simulink model "Nadir_Pointing"  (R2023b)
settings: Solver=VariableStepAuto  StartTime=0.0  StopTime=10.0  RelTol=1e-3
values from neighbouring files (symbols this model uses):
  a = 7259    [Group_51.m]
  a_sun = 149.60e6    (= 149600000)    [Group_51.m]
  ARW = (((arw*pi/180)/(sqrt(n_t)))^2)*n_t    [Group_51.m]
  Beta_CMG = acos(dot([1;0;0],uv_pyr))    [Group_51.m]
  delta_0_P = SM.delta_g_SM(end,:)    [Group_51.m]
  e = 0.001    [Group_51.m]
  e_sun = 0.0167086    [Group_51.m]
  eps_b = 11.5*pi/180    (= 0.200712863979)    [Group_51.m]
  eps_sun = deg2rad(23.45)    [Group_51.m]
  f0_P = SM.Theta_SM(end,1)    [Group_51.m]
  g_1_0 = -29404.8    [Group_51.m]
  g_1_1 = -1450.9    [Group_51.m]
  Gain_G = eye(3,3)    [Group_51.m]
  h_1_1 = 4653.5    [Group_51.m]
  h_r = [0.5;0.5;0.5;0.5]    [Group_51.m]
  halfrange = pi/40    (= 0.0785398163397)    [Group_51.m]
  i = deg2rad(97.27276)    [Group_51.m]
  I_tot = I+Ip_1_transp+Ip_2_transp    [Group_51.m]
  I_tot_inv = I_tot\eye(3,3)    [Group_51.m]
  IC312_P = [phi312_P;theta312_P;psi312_P]    [Group_51.m]
  jb = [0.1; 0.1;0.1]    [Group_51.m]
  k_cmg = -1    [Group_51.m]
  kdx_P = 2    [Group_51.m]
  kdy_P = 2.365    [Group_51.m]
  kdz_P = 2.1    [Group_51.m]
  kpx_SM = 0.129*0.5    (= 0.0645)    [Group_51.m]
  kpy_P = 1.4*0.5    (= 0.7)    [Group_51.m]
  kpz_P = 1*0.5    (= 0.5)    [Group_51.m]
  Miss_G = [teta_g_x;teta_g_y;teta_g_z]    [Group_51.m]
  n = sqrt(mu/ a^3)    [Group_51.m]
  n_sun = 2*pi/(365.26*24*3600)    (= 1.99096676796e-07)    [Group_51.m]
  n_t = samp_t    (= 1)    [Group_51.m]
  OM = deg2rad(90)    [Group_51.m]
  Re = astroConstants(23)    [Group_51.m]
  RRW = (((rrw*pi/180)/(sqrt(n_t)))^2)*n_t    [Group_51.m]
  samp_t = 1/samp_freq    (= 1)    [Group_51.m]
  t_sun_P = tf_D+tf_SM    (= 550)    [Group_51.m]
  w = deg2rad(0)    [Group_51.m]
  w0_P = [wx_P;wy_P;wz_P]    [Group_51.m]
  we = we/3600    (= 7.29159776389e-06)    [Group_51.m]
undefined symbols (not defined in the file or in its folder): DiscIntNeverNeededParam
libraries: matrix_library x15, vrlib x11, simulink x6, hdlsllib x2, dspswit3 x1
(part 1 of 2)
settings Model: Creator=leo-deo  LastModifiedBy=leo-deo

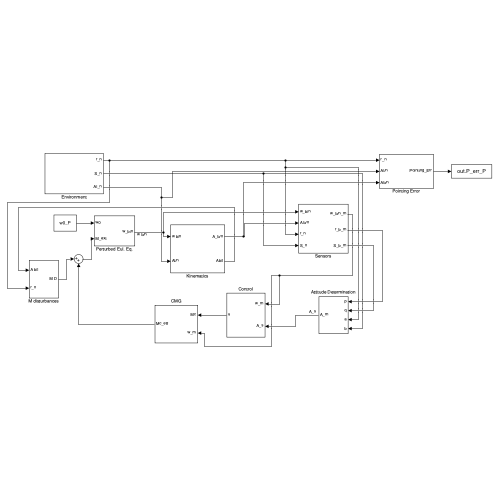
[thumbnail: Simulink's stored preview of the top-level diagram]
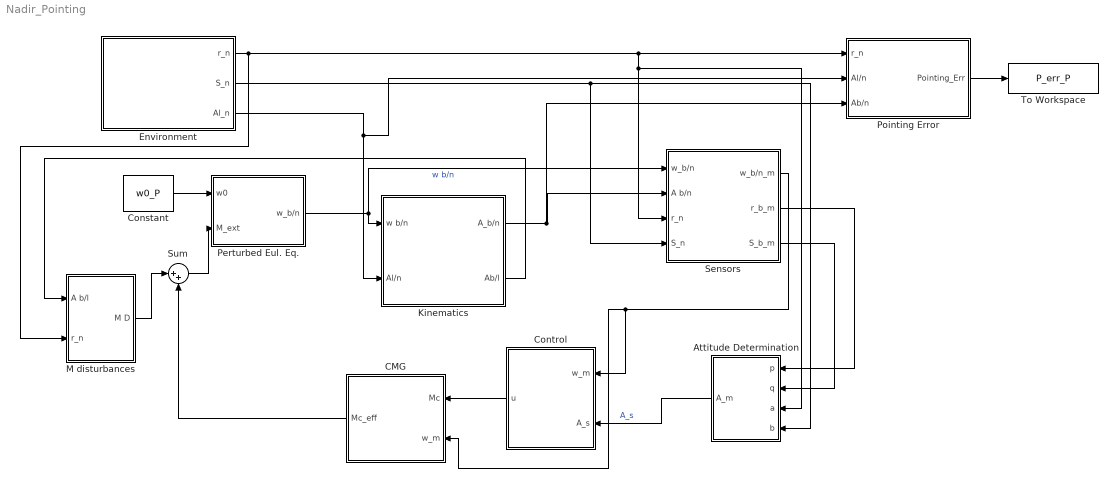
== system Nadir_Pointing ==
  Attitude Determination : Subsystem
  CMG : Subsystem
  Constant : Constant  Value=w0_P
  Control : Subsystem
  Environment : Subsystem
  Kinematics : Subsystem
  M disturbances : Subsystem
  Perturbed Eul. Eq. : Subsystem
  Pointing Error : Subsystem
  Sensors : Subsystem
  Sum : Sum  Inputs=|++
  To Workspace : ToWorkspace  VariableName=P_err_P  SampleTime=-1
  wires:
  M disturbances/1(M D) -> Sum/1
  Sensors/3(S_b_m) -> Attitude Determination/2(q)
  Kinematics/2(Ab/l) -> M disturbances/1(A b/l)
  Environment/2(S_n) -> Attitude Determination/4(b), Sensors/4(S_n)
  Sensors/1(w_b/n_m) -> Control/1(w_m), CMG/2(w_m)
  Kinematics/1(A_b/n) -> Pointing Error/3(Ab/n), Sensors/2(A b/n)
  Perturbed Eul. Eq./1(w_b/n) -> Sensors/1(w_b/n), Kinematics/1(w b/n)  "w b/n"
  Environment/3(Al_n) -> Pointing Error/2(Al/n), Kinematics/2(Al/n)
  Sum/1 -> Perturbed Eul. Eq./2(M_ext)
  Sensors/2(r_b_m) -> Attitude Determination/1(p)
  Constant/1 -> Perturbed Eul. Eq./1(w0)
  CMG/1(Mc_eff) -> Sum/2
  Control/1(u) -> CMG/1(Mc)
  Environment/1(r_n) -> M disturbances/2(r_n), Pointing Error/1(r_n), Attitude Determination/3(a), Sensors/3(r_n)
  Attitude Determination/1(A_m) -> Control/2(A_s)  "A_s"
  Pointing Error/1(Pointing_Err) -> To Workspace/1

== system Nadir_Pointing/Attitude Determination ==
  p : Inport
  q : Inport  Port=2
  a : Inport  Port=3
  b : Inport  Port=4
  Cross Product{,1..3} (4 alike) : matrix_library/Cross Product
  Matrix Concatenate : Concatenate  NumInputs=3  Mode=Multidimensional array  ConcatenateDimension=2
  Matrix Concatenate1 : Concatenate  NumInputs=3  Mode=Multidimensional array  ConcatenateDimension=2
  Normalize Vector{,1..5} (6 alike) : vrlib/Utilities/Normalize Vector  maxzero=0
  Product : Product  Multiplication=Matrix(*)
  Transpose : Math  Operator=transpose
  Zero-Order Hold : ZeroOrderHold  SampleTime=samp_t
  Zero-Order Hold1 : ZeroOrderHold  SampleTime=samp_t
  A_m : Outport
  wires:
  Matrix Concatenate1/1 -> Transpose/1
  Cross Product/1 -> Normalize Vector4/1
  Normalize Vector3/1 -> Matrix Concatenate1/3  "v3"
  Cross Product3/1 -> Normalize Vector3/1
  Product/1 -> A_m/1
  Cross Product1/1 -> Normalize Vector5/1
  Transpose/1 -> Product/2
  Matrix Concatenate/1 -> Product/1
  Normalize Vector2/1 -> Matrix Concatenate1/2, Cross Product3/2  "v2"
  Normalize Vector4/1 -> Matrix Concatenate/2, Cross Product1/2  "s2"
  q/1 -> Cross Product/2
  Cross Product2/1 -> Normalize Vector2/1
  p/1 -> Cross Product/1, Matrix Concatenate/1, Cross Product1/1  "s1"
  a/1 -> Zero-Order Hold/1
  Normalize Vector/1 -> Matrix Concatenate1/1, Cross Product3/1, Cross Product2/1  "v1"
  b/1 -> Zero-Order Hold1/1
  Normalize Vector1/1 -> Cross Product2/2
  Zero-Order Hold/1 -> Normalize Vector/1
  Zero-Order Hold1/1 -> Normalize Vector1/1
  Normalize Vector5/1 -> Matrix Concatenate/3

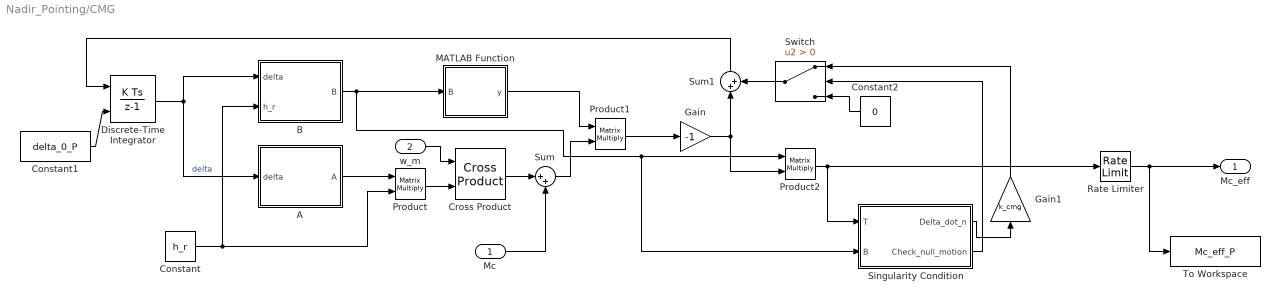
== system Nadir_Pointing/CMG ==
  Mc : Inport
  w_m : Inport  Port=2
  A : Subsystem
  B : Subsystem
  Constant : Constant  Value=h_r
  Constant1 : Constant  Value=delta_0_P
  Constant2 : Constant  Value=0
  Cross Product : matrix_library/Cross Product
  Discrete-Time Integrator : DiscreteIntegrator  InitialConditionSource=external  SampleTime=-1  ICPrevOutput=DiscIntNeverNeededParam  ICPrevScaledInput=DiscIntNeverNeededParam
  Gain : Gain  Gain=-1
  Gain1 : Gain  Gain=k_cmg
  MATLAB Function : MATLAB Function  TreatAsAtomicUnit=on
  Product : Product  Multiplication=Matrix(*)
  Product1 : Product  Multiplication=Matrix(*)
  Product2 : Product  Multiplication=Matrix(*)
  Rate Limiter : RateLimiter  RisingSlewLimit=samp_t  FallingSlewLimit=-samp_t
  Singularity Condition : Subsystem
  Sum : Sum  Inputs=|++
  Sum1 : Sum  Inputs=|++
  Switch : Switch  Criteria=u2 > Threshold  SaturateOnIntegerOverflow=off  InputSameDT=off
  To Workspace : ToWorkspace  VariableName=Mc_eff_P  SampleTime=-1
  Mc_eff : Outport
  wires:
  Rate Limiter/1 -> To Workspace/1, Mc_eff/1
  MATLAB Function/1(y) -> Product1/1
  Discrete-Time Integrator/1 -> B/1(delta), A/1(delta)  "delta"
  w_m/1 -> Cross Product/1
  Cross Product/1 -> Sum/1
  Sum/1 -> Product1/2
  Product1/1 -> Gain/1
  Constant/1 -> B/2(h_r), Product/2
  B/1(B) -> MATLAB Function/1(B), Singularity Condition/2(B), Product2/1
  Product/1 -> Cross Product/2
  A/1(A) -> Product/1
  Gain/1 -> Sum1/1, Product2/2
  Constant1/1 -> Discrete-Time Integrator/2
  Product2/1 -> Rate Limiter/1, Singularity Condition/1(T)
  Sum1/1 -> Discrete-Time Integrator/1
  Switch/1 -> Sum1/2
  Constant2/1 -> Switch/3
  Singularity Condition/2(Check_null_motion) -> Switch/2
  Mc/1 -> Sum/2
  Singularity Condition/1(Delta_dot_n) -> Gain1/1
  Gain1/1 -> Switch/1

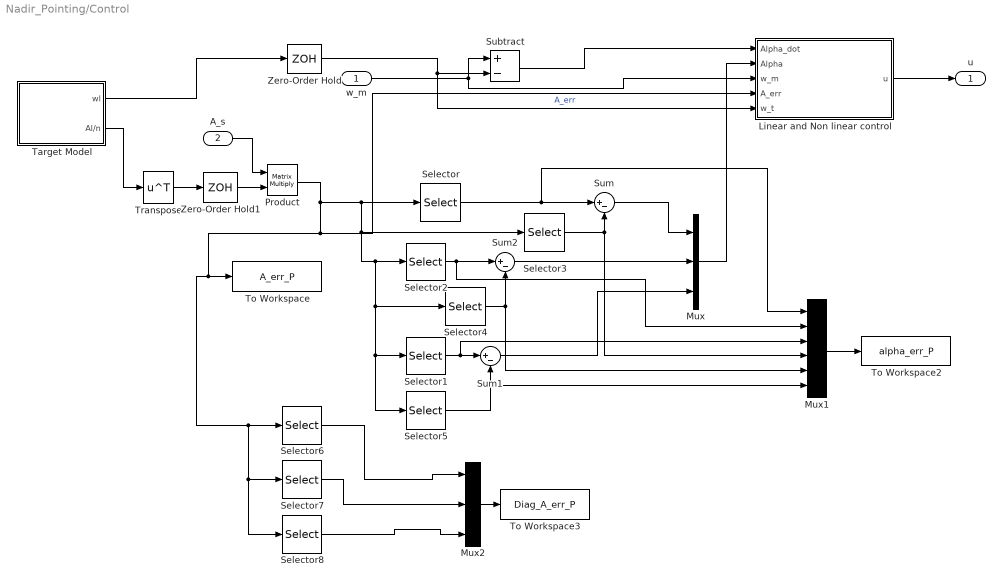
== system Nadir_Pointing/Control ==
  w_m : Inport
  A_s : Inport  Port=2
  Linear and Non linear control : Subsystem
  Mux : Mux  Inputs=3
  Mux1 : Mux  Inputs=6
  Mux2 : Mux  Inputs=3
  Product : Product  Multiplication=Matrix(*)
  Selector : Selector  NumberOfDimensions=2  InputPortWidth=3  IndexOptions=Index vector (dialog),Index vector (dialog)  Indices=2,3  OutputSizes=1,1
  Selector1 : Selector  NumberOfDimensions=2  InputPortWidth=3  IndexOptions=Index vector (dialog),Index vector (dialog)  Indices=1,2  OutputSizes=1,1
  Selector2 : Selector  NumberOfDimensions=2  InputPortWidth=3  IndexOptions=Index vector (dialog),Index vector (dialog)  Indices=3,1  OutputSizes=1,1
  Selector3 : Selector  NumberOfDimensions=2  InputPortWidth=3  IndexOptions=Index vector (dialog),Index vector (dialog)  Indices=3,2  OutputSizes=1,1
  Selector4 : Selector  NumberOfDimensions=2  InputPortWidth=3  IndexOptions=Index vector (dialog),Index vector (dialog)  Indices=1,3  OutputSizes=1,1
  Selector5 : Selector  NumberOfDimensions=2  InputPortWidth=3  IndexOptions=Index vector (dialog),Index vector (dialog)  Indices=2,1  OutputSizes=1,1
  Selector6 : Selector  NumberOfDimensions=2  InputPortWidth=3  IndexOptions=Index vector (dialog),Index vector (dialog)  Indices=1,1  OutputSizes=1,1
  Selector7 : Selector  NumberOfDimensions=2  InputPortWidth=3  IndexOptions=Index vector (dialog),Index vector (dialog)  Indices=2,2  OutputSizes=1,1
  Selector8 : Selector  NumberOfDimensions=2  InputPortWidth=3  IndexOptions=Index vector (dialog),Index vector (dialog)  Indices=3,3  OutputSizes=1,1
  Subtract : Sum  Inputs=+-
  Sum : Sum  Inputs=|+-
  Sum1 : Sum  Inputs=|+-
  Sum2 : Sum  Inputs=|+-
  Target Model : Subsystem
  To Workspace : ToWorkspace  VariableName=A_err_P  SampleTime=-1
  To Workspace2 : ToWorkspace  VariableName=alpha_err_P  SampleTime=-1
  To Workspace3 : ToWorkspace  VariableName=Diag_A_err_P  SampleTime=-1
  Transpose : Math  Operator=transpose
  Zero-Order Hold : ZeroOrderHold  SampleTime=samp_t
  Zero-Order Hold1 : ZeroOrderHold  SampleTime=samp_t
  u : Outport
  wires:
  A_s/1 -> Product/1
  Target Model/2(Al/n) -> Transpose/1
  Subtract/1 -> Linear and Non linear control/1(Alpha_dot)
  w_m/1 -> Linear and Non linear control/3(w_m), Subtract/1
  Product/1 -> Selector3/1, Selector4/1, Selector5/1, Selector1/1, Selector2/1, Selector/1, To Workspace/1, Selector8/1, Selector7/1, Selector6/1, Linear and Non linear control/4(A_err)  "A_err"
  Linear and Non linear control/1(u) -> u/1
  Selector/1 -> Mux1/1, Sum/1
  Selector2/1 -> Mux1/2, Sum2/1
  Selector1/1 -> Mux1/3, Sum1/1
  Selector3/1 -> Mux1/4, Sum/2
  Sum/1 -> Mux/1
  Mux/1 -> Linear and Non linear control/2(Alpha)
  Selector4/1 -> Sum2/2, Mux1/5
  Sum2/1 -> Mux/2
  Selector5/1 -> Mux1/6, Sum1/2
  Sum1/1 -> Mux/3
  Mux1/1 -> To Workspace2/1
  Transpose/1 -> Zero-Order Hold1/1
  Selector7/1 -> Mux2/2
  Selector8/1 -> Mux2/3
  Mux2/1 -> To Workspace3/1
  Selector6/1 -> Mux2/1
  Target Model/1(wl) -> Zero-Order Hold/1
  Zero-Order Hold/1 -> Linear and Non linear control/5(w_t), Subtract/2
  Zero-Order Hold1/1 -> Product/2

== system Nadir_Pointing/Environment ==
  A l/n for elliptical orbit : Subsystem
  Clock : Clock
  Kep 2bp : Subsystem
  "Sn " : Subsystem
  To Workspace : ToWorkspace  VariableName=t_P  SampleTime=-1
  r_n : Outport
  S_n : Outport  Port=2
  Al_n : Outport  Port=3
  wires:
  Kep 2bp/1(r_n) -> r_n/1
  "Sn "/1(Sn) -> S_n/1
  A l/n for elliptical orbit/1(Al/n) -> Al_n/1
  Clock/1 -> To Workspace/1
  A l/n for elliptical orbit/2(Theta) -> Kep 2bp/1(Theta)

== system Nadir_Pointing/Kinematics ==
  w b/n : Inport
  Al/n : Inport  Port=2
  Euler Angles : Subsystem
  Product2 : Product  Multiplication=Matrix(*)
  Subsystem : Subsystem
  To Workspace : ToWorkspace  VariableName=A_bn_P  SampleTime=-1
  Transpose1 : Math  Operator=transpose
  A_b/n : Outport
  Ab/l : Outport  Port=2
  wires:
  w b/n/1 -> Euler Angles/1(w_b)
  Al/n/1 -> Transpose1/1
  Transpose1/1 -> Product2/2
  Product2/1 -> Ab/l/1  "Ab/l"
  Euler Angles/1(A_b/n) -> Product2/1, To Workspace/1, A_b/n/1
  Euler Angles/2(Ang_312) -> Subsystem/1(Ang_312)
  Euler Angles/3(Ang_313) -> Subsystem/2(Ang_313)
  Euler Angles/4(T-F) -> Subsystem/3(T-F)

== system Nadir_Pointing/M disturbances ==
  A b/l : Inport
  r_n : Inport  Port=2
  M of B : Subsystem
  M of G G : Subsystem
  Sum : Sum  Inputs=||+||+||
  M D : Outport
  wires:
  Sum/1 -> M D/1
  A b/l/1 -> M of B/1(A b/n), M of G G/1(Ab/l)
  M of G G/1(M_G_G) -> Sum/2
  M of B/1(M B) -> Sum/1
  r_n/1 -> M of B/2(r_n)

== system Nadir_Pointing/Perturbed Eul. Eq. ==
  w0 : Inport
  M_ext : Inport  Port=2
  Constant2 : Constant  Value=I_tot
  Constant3 : Constant  Value=I_tot_inv
  Cross Product : matrix_library/Cross Product
  Integrator1 : Integrator  InitialConditionSource=external  AbsoluteTolerance=1e-10
  Product : Product  Multiplication=Matrix(*)
  Product1 : Product  Multiplication=Matrix(*)
  Product2 : Product  Multiplication=Matrix(*)
  Sum : Sum  Inputs=|-+
  To Workspace : ToWorkspace  VariableName=w_b_P  SampleTime=-1
  w_b/n : Outport
  wires:
  Constant2/1 -> Product/1
  Product/1 -> Cross Product/2
  Product2/1 -> Sum/2
  Sum/1 -> Integrator1/1
  Constant3/1 -> Product2/1, Product1/1
  Cross Product/1 -> Product1/2
  Integrator1/1 -> Cross Product/1, Product/2, To Workspace/1, w_b/n/1
  Product1/1 -> Sum/1
  w0/1 -> Integrator1/2
  M_ext/1 -> Product2/2

== system Nadir_Pointing/Pointing Error ==
  r_n : Inport
  Al/n : Inport  Port=2
  Ab/n : Inport  Port=3
  Acos : Trigonometry  Operator=acos
  Dot Product : DotProduct  OutDataTypeStr=Inherit: Inherit via internal rule
  Normalize Vector : vrlib/Utilities/Normalize Vector  maxzero=0
  Normalize Vector1 : vrlib/Utilities/Normalize Vector  maxzero=0
  Product : Product  Multiplication=Matrix(*)
  Product1 : Product  Multiplication=Matrix(*)
  Scope : Scope
  Pointing_Err : Outport
  wires:
  Ab/n/1 -> Product1/1
  Al/n/1 -> Product/1
  Normalize Vector/1 -> Dot Product/2
  Product1/1 -> Normalize Vector/1
  Dot Product/1 -> Acos/1
  r_n/1 -> Product/2, Product1/2
  Normalize Vector1/1 -> Dot Product/1
  Product/1 -> Normalize Vector1/1
  Acos/1 -> Scope/1, Pointing_Err/1

== system Nadir_Pointing/Sensors ==
  w_b/n : Inport
  A b/n : Inport  Port=2
  r_n : Inport  Port=3
  S_n : Inport  Port=4
  Clock : Clock
  Gyroscopic Sensor : Subsystem
  Horizon Sensor1 : Subsystem
  Normalize Vector : vrlib/Utilities/Normalize Vector  maxzero=0
  Normalize Vector1 : vrlib/Utilities/Normalize Vector  maxzero=0
  Product : Product  Multiplication=Matrix(*)
  Product1 : Product  Multiplication=Matrix(*)
  Sun Sensor1 : Subsystem
  To Workspace : ToWorkspace  VariableName=t_s_P  SampleTime=-1
  Zero-Order Hold : ZeroOrderHold  SampleTime=samp_t
  w_b/n_m : Outport
  r_b_m : Outport  Port=2
  S_b_m : Outport  Port=3
  wires:
  S_n/1 -> Product1/2
  Product/1 -> Normalize Vector/1
  A b/n/1 -> Product/1, Product1/1
  r_n/1 -> Product/2
  w_b/n/1 -> Gyroscopic Sensor/1(w_b/n)
  Sun Sensor1/1(S_b_m) -> S_b_m/1  "s3"
  Normalize Vector1/1 -> Sun Sensor1/1(S_b)  "s3"
  Product1/1 -> Normalize Vector1/1
  Gyroscopic Sensor/1(w_b/n_m) -> w_b/n_m/1
  Normalize Vector/1 -> Horizon Sensor1/1(r_b)  "s3"
  Horizon Sensor1/1(r_b_m) -> r_b_m/1  "s3"
  Clock/1 -> Zero-Order Hold/1
  Zero-Order Hold/1 -> To Workspace/1

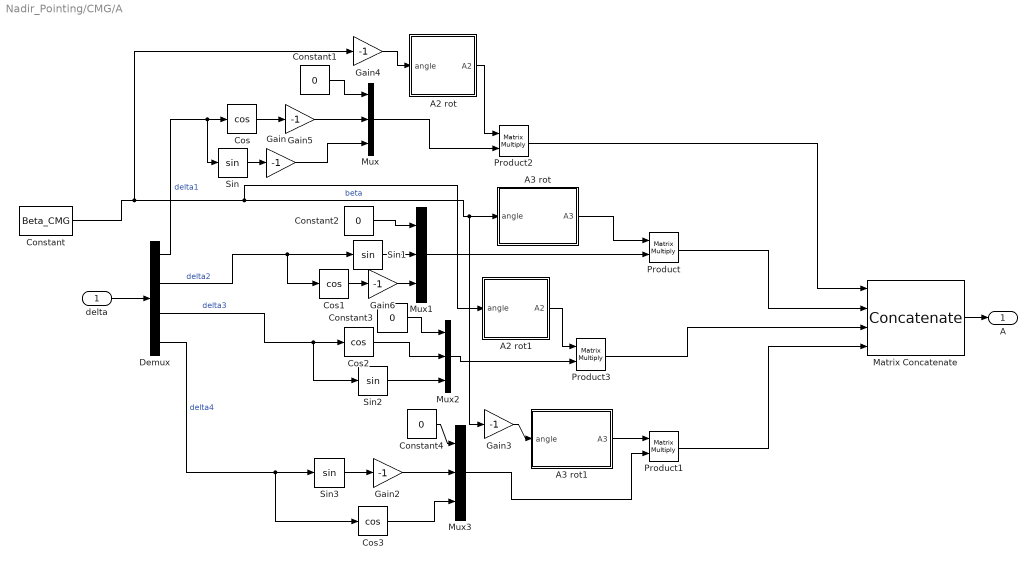
== system Nadir_Pointing/CMG/A ==
  delta : Inport
  A2 rot : Subsystem
  A2 rot1 : Subsystem
  A3 rot : Subsystem
  A3 rot1 : Subsystem
  Constant : Constant  Value=Beta_CMG
  Constant{1..4} (4 alike) : Constant  Value=0
  Cos{,1..3} (4 alike) : Trigonometry  Operator=cos
  Demux : Demux
  Gain{,2..6} (6 alike) : Gain  Gain=-1
  Matrix Concatenate : Concatenate  NumInputs=4  Mode=Multidimensional array  ConcatenateDimension=2
  Mux{,1..3} (4 alike) : Mux  Inputs=3
  Product{,1..3} (4 alike) : Product  Multiplication=Matrix(*)
  Sin{,1..3} (4 alike) : Trigonometry
  A : Outport
  wires:
  Constant4/1 -> Mux3/1
  Constant2/1 -> Mux1/1
  Sin3/1 -> Gain2/1
  Sin/1 -> Gain/1
  delta/1 -> Demux/1
  Demux/1 -> Sin/1, Cos/1  "delta1"
  Gain/1 -> Mux/3
  Constant1/1 -> Mux/1
  Constant3/1 -> Mux2/1
  Sin1/1 -> Mux1/2
  Demux/2 -> Cos1/1, Sin1/1  "delta2"
  Cos3/1 -> Mux3/3
  Gain2/1 -> Mux3/2
  Demux/4 -> Cos3/1, Sin3/1  "delta4"
  Mux1/1 -> Product/2
  Constant/1 -> Gain4/1, A2 rot1/1(angle), Gain3/1, A3 rot/1(angle)  "beta"
  A3 rot/1(A3) -> Product/1
  Product/1 -> Matrix Concatenate/2
  Gain3/1 -> A3 rot1/1(angle)
  A3 rot1/1(A3) -> Product1/1
  Mux3/1 -> Product1/2
  Product1/1 -> Matrix Concatenate/4
  A2 rot/1(A2) -> Product2/1
  Mux/1 -> Product2/2
  Gain4/1 -> A2 rot/1(angle)
  Product2/1 -> Matrix Concatenate/1
  Mux2/1 -> Product3/2
  Product3/1 -> Matrix Concatenate/3
  A2 rot1/1(A2) -> Product3/1
  Matrix Concatenate/1 -> A/1
  Gain5/1 -> Mux/2
  Cos/1 -> Gain5/1
  Gain6/1 -> Mux1/3
  Cos1/1 -> Gain6/1
  Sin2/1 -> Mux2/3
  Cos2/1 -> Mux2/2
  Demux/3 -> Sin2/1, Cos2/1  "delta3"

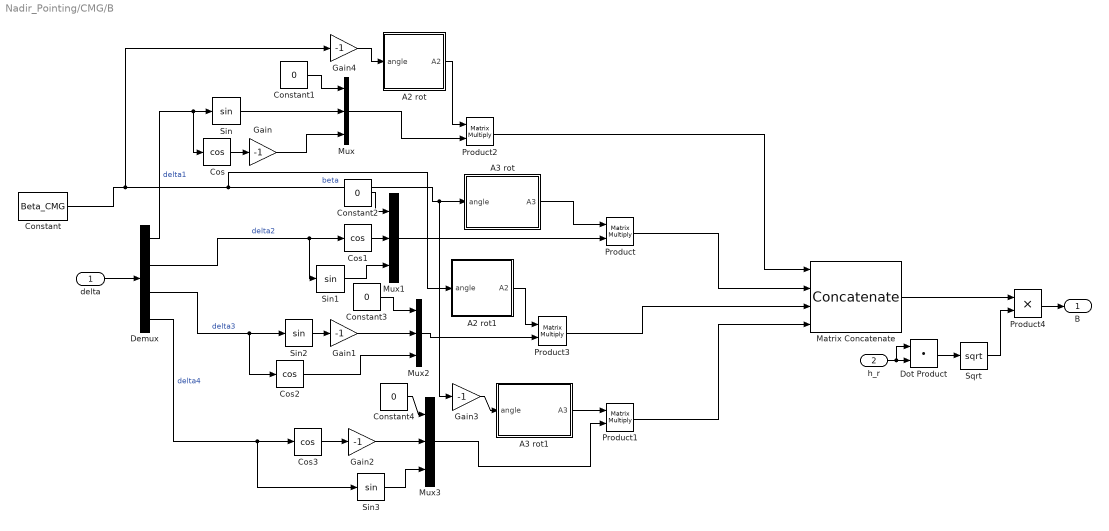
== system Nadir_Pointing/CMG/B ==
  delta : Inport
  h_r : Inport  Port=2
  A2 rot : Subsystem
  A2 rot1 : Subsystem
  A3 rot : Subsystem
  A3 rot1 : Subsystem
  Constant : Constant  Value=Beta_CMG
  Constant{1..4} (4 alike) : Constant  Value=0
  Cos{,1..3} (4 alike) : Trigonometry  Operator=cos
  Demux : Demux
  Dot Product : DotProduct  OutDataTypeStr=Inherit: Inherit via internal rule
  Gain{,1..4} (5 alike) : Gain  Gain=-1
  Matrix Concatenate : Concatenate  NumInputs=4  Mode=Multidimensional array  ConcatenateDimension=2
  Mux{,1..3} (4 alike) : Mux  Inputs=3
  Product{,1..3} (4 alike) : Product  Multiplication=Matrix(*)
  Product4 : Product
  Sin{,1..3} (4 alike) : Trigonometry
  Sqrt : Sqrt
  B : Outport
  wires:
  Constant4/1 -> Mux3/1
  Sin1/1 -> Mux1/3
  Constant2/1 -> Mux1/1
  Cos3/1 -> Gain2/1
  Cos/1 -> Gain/1
  delta/1 -> Demux/1
  Demux/1 -> Cos/1, Sin/1  "delta1"
  Gain/1 -> Mux/3
  Gain1/1 -> Mux2/2
  Constant1/1 -> Mux/1
  Constant3/1 -> Mux2/1
  Cos1/1 -> Mux1/2
  Demux/2 -> Cos1/1, Sin1/1  "delta2"
  Sin3/1 -> Mux3/3
  Cos2/1 -> Mux2/3
  Gain2/1 -> Mux3/2
  Sin/1 -> Mux/2
  Demux/4 -> Sin3/1, Cos3/1  "delta4"
  Sin2/1 -> Gain1/1
  Demux/3 -> Cos2/1, Sin2/1  "delta3"
  Mux1/1 -> Product/2
  Constant/1 -> Gain4/1, A2 rot1/1(angle), Gain3/1, A3 rot/1(angle)  "beta"
  A3 rot/1(A3) -> Product/1
  Product/1 -> Matrix Concatenate/2
  Gain3/1 -> A3 rot1/1(angle)
  A3 rot1/1(A3) -> Product1/1
  Mux3/1 -> Product1/2
  Product1/1 -> Matrix Concatenate/4
  A2 rot/1(A2) -> Product2/1
  Mux/1 -> Product2/2
  Gain4/1 -> A2 rot/1(angle)
  Product2/1 -> Matrix Concatenate/1
  Mux2/1 -> Product3/2
  Product3/1 -> Matrix Concatenate/3
  A2 rot1/1(A2) -> Product3/1
  Product4/1 -> B/1
  Matrix Concatenate/1 -> Product4/1
  h_r/1 -> Dot Product/1, Dot Product/2
  Dot Product/1 -> Sqrt/1
  Sqrt/1 -> Product4/2

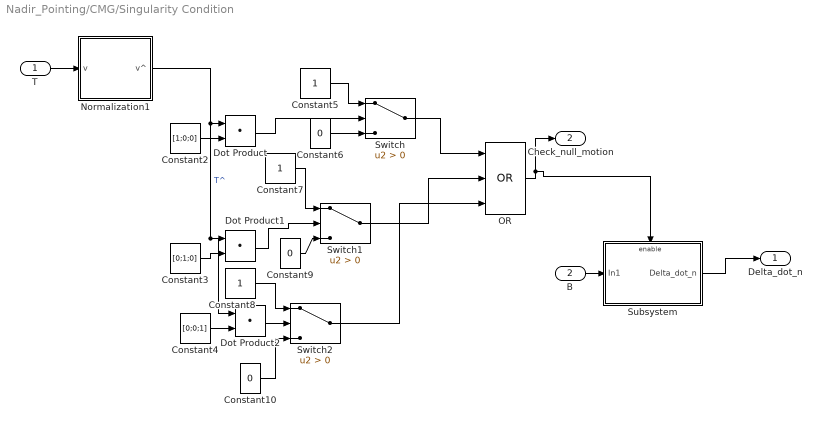
== system Nadir_Pointing/CMG/Singularity Condition ==
  T : Inport
  B : Inport  Port=2
  Constant10 : Constant  Value=0
  Constant2 : Constant  Value=[1;0;0]
  Constant3 : Constant  Value=[0;1;0]
  Constant4 : Constant  Value=[0;0;1]
  Constant5 : Constant
  Constant6 : Constant  Value=0
  Constant7 : Constant
  Constant8 : Constant
  Constant9 : Constant  Value=0
  Dot Product : DotProduct  OutDataTypeStr=Inherit: Inherit via internal rule
  Dot Product1 : DotProduct  OutDataTypeStr=Inherit: Inherit via internal rule
  Dot Product2 : DotProduct  OutDataTypeStr=Inherit: Inherit via internal rule
  Normalization1 : Subsystem
  OR : Logic  Operator=OR  Inputs=3  IconShape=distinctive  AllPortsSameDT=off  OutDataTypeStr=boolean
  Subsystem : Subsystem
  Switch : Switch  Criteria=u2 > Threshold  SaturateOnIntegerOverflow=off  InputSameDT=off
  Switch1 : Switch  Criteria=u2 > Threshold  SaturateOnIntegerOverflow=off  InputSameDT=off
  Switch2 : Switch  Criteria=u2 > Threshold  SaturateOnIntegerOverflow=off  InputSameDT=off
  Delta_dot_n : Outport
  Check_null_motion : Outport  Port=2
  wires:
  Constant2/1 -> Dot Product/2
  T/1 -> Normalization1/1(v)
  Constant3/1 -> Dot Product1/2
  Switch2/1 -> OR/3
  Constant9/1 -> Switch1/3
  Dot Product1/1 -> Switch1/2
  Switch1/1 -> OR/2
  Normalization1/1(v^) -> Dot Product2/1, Dot Product1/1, Dot Product/1  "T^"
  Dot Product2/1 -> Switch2/2
  Dot Product/1 -> Switch/2
  Constant8/1 -> Switch2/1
  Switch/1 -> OR/1
  Constant5/1 -> Switch/1
  Constant4/1 -> Dot Product2/2
  Constant6/1 -> Switch/3
  Constant7/1 -> Switch1/1
  Constant10/1 -> Switch2/3
  OR/1 -> Subsystem/Enable, Check_null_motion/1
  Subsystem/1(Delta_dot_n) -> Delta_dot_n/1
  B/1 -> Subsystem/1(In1)

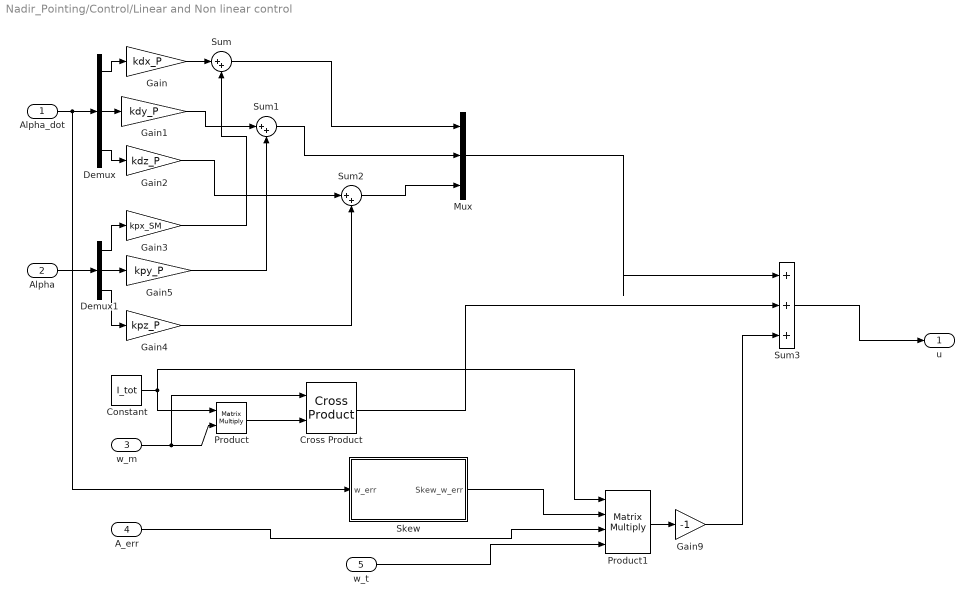
== system Nadir_Pointing/Control/Linear and Non linear control ==
  Alpha_dot : Inport
  Alpha : Inport  Port=2
  w_m : Inport  Port=3
  A_err : Inport  Port=4
  w_t : Inport  Port=5
  Constant : Constant  Value=I_tot
  Cross Product : matrix_library/Cross Product
  Demux : Demux  Outputs=3
  Demux1 : Demux  Outputs=3
  Gain : Gain  Gain=kdx_P
  Gain1 : Gain  Gain=kdy_P
  Gain2 : Gain  Gain=kdz_P
  Gain3 : Gain  Gain=kpx_SM
  Gain4 : Gain  Gain=kpz_P
  Gain5 : Gain  Gain=kpy_P
  Gain9 : Gain  Gain=-1
  Mux : Mux  Inputs=3
  Product : Product  Multiplication=Matrix(*)
  Product1 : Product  Inputs=4  Multiplication=Matrix(*)
  Skew : Subsystem
  Sum : Sum  Inputs=|++
  Sum1 : Sum  Inputs=|++
  Sum2 : Sum  Inputs=|++
  Sum3 : Sum  Inputs=|+++
  u : Outport
  wires:
  Alpha_dot/1 -> Skew/1(w_err), Demux/1
  Alpha/1 -> Demux1/1
  Demux/1 -> Gain/1
  Demux/2 -> Gain1/1
  Gain/1 -> Sum/1
  Sum/1 -> Mux/1
  Gain2/1 -> Sum2/1
  Gain1/1 -> Sum1/1
  Demux1/1 -> Gain3/1
  Demux1/2 -> Gain5/1
  Demux1/3 -> Gain4/1
  Sum1/1 -> Mux/2
  Sum2/1 -> Mux/3
  Gain3/1 -> Sum/2
  Gain5/1 -> Sum1/2
  Gain4/1 -> Sum2/2
  Constant/1 -> Product/1, Product1/1
  w_m/1 -> Cross Product/1, Product/2
  Product/1 -> Cross Product/2
  Demux/3 -> Gain2/1
  w_t/1 -> Product1/4
  Skew/1(Skew_w_err) -> Product1/2
  Product1/1 -> Gain9/1
  Sum3/1 -> u/1
  Mux/1 -> Sum3/1
  Cross Product/1 -> Sum3/2
  Gain9/1 -> Sum3/3
  A_err/1 -> Product1/3

== system Nadir_Pointing/Control/Target Model ==
  Arg. of perigee : Constant  Value=w
  Constant : Constant  Value=[0;0;1]
  Constant3 : Constant  Value=f0_P
  Inclination : Constant  Value=i
  Product : Product
  RAAN : Constant  Value=OM
  Subsystem : Subsystem
  Subsystem1 : Subsystem
  Sum : Sum  Inputs=|++
  wl : Outport
  Al/n : Outport  Port=2
  wires:
  Sum/1 -> Subsystem1/3(w+f)
  Constant/1 -> Product/2
  Inclination/1 -> Subsystem1/2(i)
  Subsystem/2(teta_dot) -> Product/1
  Product/1 -> wl/1
  Constant3/1 -> Subsystem/1(True Anomaly0)
  Arg. of perigee/1 -> Sum/1
  RAAN/1 -> Subsystem1/1(OM)
  Subsystem1/1(A313) -> Al/n/1
  Subsystem/1(theta) -> Sum/2  "true anomaly"

== system Nadir_Pointing/Environment/A l//n for elliptical orbit ==
  Arg. of perigee : Constant  Value=w
  Constant : Constant  Value=[0;0;1]
  Constant3 : Constant  Value=f0_P
  Inclination : Constant  Value=i
  Product : Product
  RAAN : Constant  Value=OM
  Subsystem : Subsystem
  Subsystem1 : Subsystem
  Sum : Sum  Inputs=|++
  To Workspace : ToWorkspace  VariableName=Theta_dot_P  SampleTime=-1
  To Workspace1 : ToWorkspace  VariableName=Theta_P  SampleTime=-1
  Al/n : Outport
  Theta : Outport  Port=2
  wires:
  Constant3/1 -> Subsystem/1(True Anomaly0)
  Constant/1 -> Product/2
  RAAN/1 -> Subsystem1/1(OM)
  Inclination/1 -> Subsystem1/2(i)
  Arg. of perigee/1 -> Sum/1
  Sum/1 -> Subsystem1/3(w+f)
  Subsystem/1(theta) -> To Workspace1/1, Sum/2, Theta/1  "true anomaly"
  Subsystem/2(teta_dot) -> Product/1
  Subsystem1/1(A313) -> Al/n/1
  Product/1 -> To Workspace/1

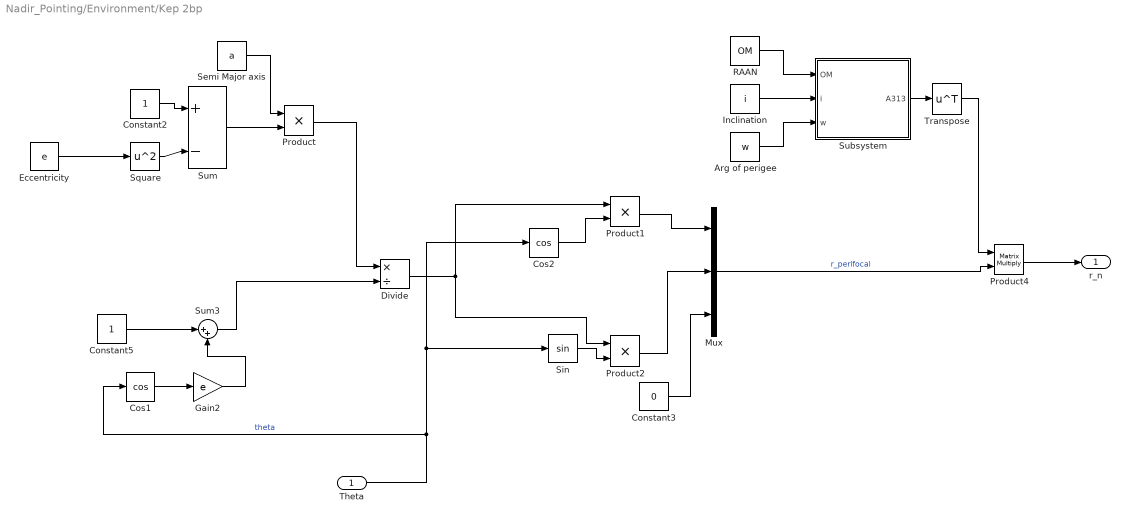
== system Nadir_Pointing/Environment/Kep 2bp ==
  Theta : Inport
  Arg of perigee : Constant  Value=w
  Constant2 : Constant
  Constant3 : Constant  Value=0
  Constant5 : Constant
  Cos1 : Trigonometry  Operator=cos
  Cos2 : Trigonometry  Operator=cos
  Divide : Product  Inputs=*/
  Eccentricity : Constant  Value=e
  Gain2 : Gain  Gain=e
  Inclination : Constant  Value=i
  Mux : Mux  Inputs=3
  Product : Product
  Product1 : Product
  Product2 : Product
  Product4 : Product  Multiplication=Matrix(*)
  RAAN : Constant  Value=OM
  Semi Major axis : Constant  Value=a
  Sin : Trigonometry
  Square : Math  Operator=square
  Subsystem : Subsystem
  Sum : Sum  Inputs=|+-
  Sum3 : Sum  Inputs=|++
  Transpose : Math  Operator=transpose
  r_n : Outport
  wires:
  Cos2/1 -> Product1/2
  Eccentricity/1 -> Square/1
  Sum/1 -> Product/2
  RAAN/1 -> Subsystem/1(OM)
  Product1/1 -> Mux/1
  Cos1/1 -> Gain2/1
  Constant2/1 -> Sum/1
  Product/1 -> Divide/1
  Constant5/1 -> Sum3/1
  Sin/1 -> Product2/2
  Theta/1 -> Cos1/1, Sin/1, Cos2/1  "theta"
  Square/1 -> Sum/2
  Gain2/1 -> Sum3/2
  Sum3/1 -> Divide/2
  Product2/1 -> Mux/2
  Semi Major axis/1 -> Product/1
  Divide/1 -> Product2/1, Product1/1
  Subsystem/1(A313) -> Transpose/1
  Arg of perigee/1 -> Subsystem/3(w)
  Product4/1 -> r_n/1
  Inclination/1 -> Subsystem/2(i)
  Constant3/1 -> Mux/3
  Mux/1 -> Product4/2  "r_perifocal"
  Transpose/1 -> Product4/1

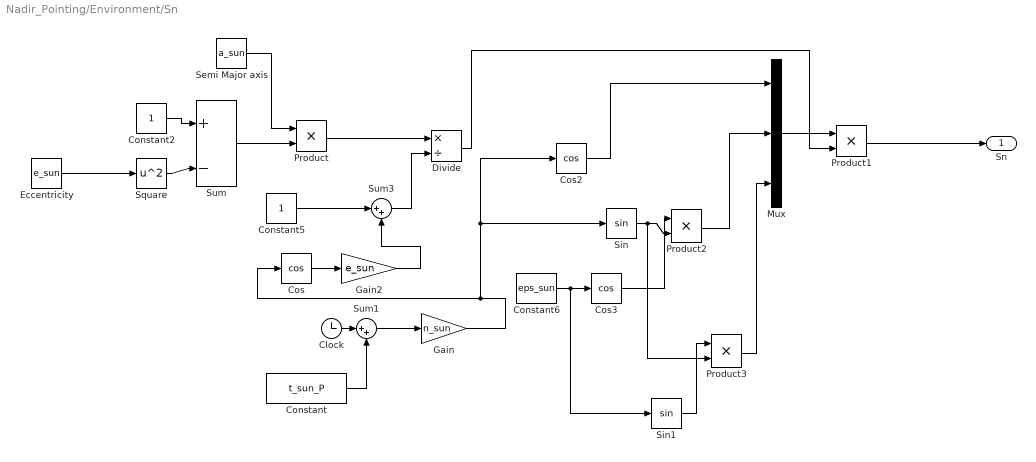
== system Nadir_Pointing/Environment/Sn  ==
  Clock : Clock
  Constant : Constant  Value=t_sun_P
  Constant2 : Constant
  Constant5 : Constant
  Constant6 : Constant  Value=eps_sun
  Cos : Trigonometry  Operator=cos
  Cos2 : Trigonometry  Operator=cos
  Cos3 : Trigonometry  Operator=cos
  Divide : Product  Inputs=*/
  Eccentricity : Constant  Value=e_sun
  Gain : Gain  Gain=n_sun
  Gain2 : Gain  Gain=e_sun
  Mux : Mux  Inputs=3
  Product{,1..3} (4 alike) : Product
  Semi Major axis : Constant  Value=a_sun
  Sin : Trigonometry
  Sin1 : Trigonometry
  Square : Math  Operator=square
  Sum : Sum  Inputs=|+-
  Sum1 : Sum  Inputs=|++
  Sum3 : Sum  Inputs=|++
  Sn : Outport
  wires:
  Constant6/1 -> Sin1/1, Cos3/1
  Sum3/1 -> Divide/2
  Cos2/1 -> Mux/1
  Constant5/1 -> Sum3/1
  Product2/1 -> Mux/2
  Product/1 -> Divide/1
  Gain2/1 -> Sum3/2
  Product3/1 -> Mux/3
  Sum/1 -> Product/2
  Eccentricity/1 -> Square/1
  Semi Major axis/1 -> Product/1
  Constant2/1 -> Sum/1
  Sin/1 -> Product3/2, Product2/2
  Gain/1 -> Sin/1, Cos2/1, Cos/1
  Square/1 -> Sum/2
  Cos3/1 -> Product2/1
  Sin1/1 -> Product3/1
  Mux/1 -> Product1/1
  Product1/1 -> Sn/1
  Divide/1 -> Product1/2
  Cos/1 -> Gain2/1
  Clock/1 -> Sum1/1
  Sum1/1 -> Gain/1
  Constant/1 -> Sum1/2

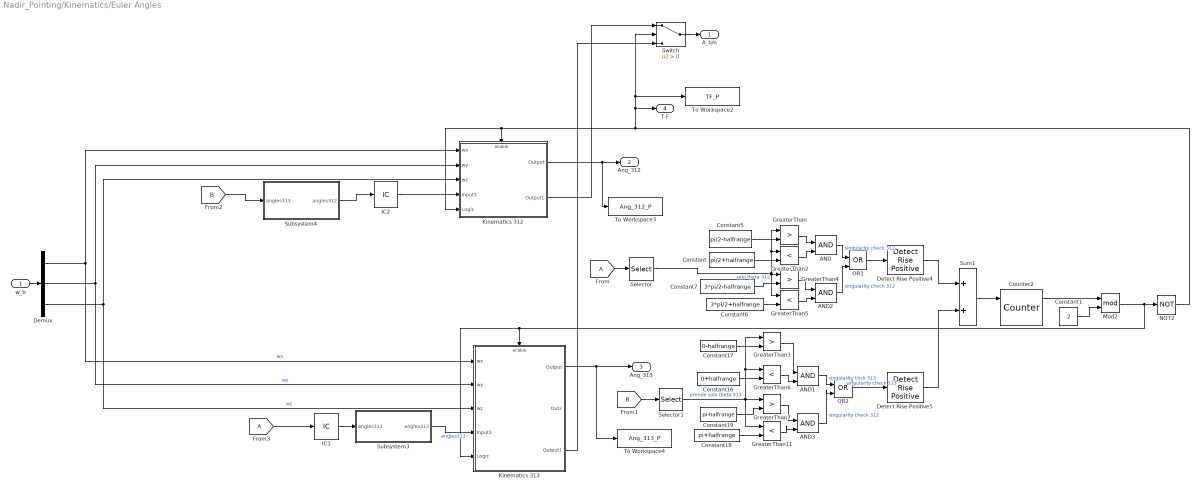
== system Nadir_Pointing/Kinematics/Euler Angles ==
  w_b : Inport
  AND{,1..3} (4 alike) : Logic  IconShape=distinctive  AllPortsSameDT=off  OutDataTypeStr=boolean
  Constant : Constant  Value=pi/2+halfrange
  Constant1 : Constant  Value=2
  Constant16 : Constant  Value=0+halfrange
  Constant17 : Constant  Value=0-halfrange
  Constant18 : Constant  Value=pi+halfrange
  Constant19 : Constant  Value=pi-halfrange
  Constant5 : Constant  Value=pi/2-halfrange
  Constant6 : Constant  Value=3*pi/2+halfrange
  Constant7 : Constant  Value=3*pi/2-halfrange
  Counter2 : dspswit3/Counter  Direction=Up  CountEvent=Rising edge  CounterSize=User defined  MaxCount=255  InitialCount=0  Output=Count and Hit  HitValue=32  ResetInput=on  SamplesPerFrame=1  Ts=1  CntDtype=double  HitDtype=Logical
  Demux : Demux  Outputs=3
  Detect Rise Positive4 : hdlsllib/Logic and Bit Operations/Detect Rise Positive  vinit=0  OutDataTypeStr=boolean
  Detect Rise Positive5 : hdlsllib/Logic and Bit Operations/Detect Rise Positive  vinit=0  OutDataTypeStr=boolean
  From : From  TagVisibility=global
  From3 : From  TagVisibility=global
  GreaterThan{,3..4,7} (4 alike) : RelationalOperator  Operator=>  OutDataTypeStr=boolean  RndMeth=Simplest  InputSameDT=off
  GreaterThan{2,5..6,11} (4 alike) : RelationalOperator  Operator=<  OutDataTypeStr=boolean  RndMeth=Simplest  InputSameDT=off
  IC1 : InitialCondition  Value=IC312_P
  IC2 : InitialCondition  Value=IC312_P
  Kinematics 312 : Subsystem
  Kinematics 313 : Subsystem
  Mod2 : Math  Operator=mod
  NOT2 : Logic  Operator=NOT  AllPortsSameDT=off  OutDataTypeStr=boolean
  OR1 : Logic  Operator=OR  IconShape=distinctive  AllPortsSameDT=off  OutDataTypeStr=boolean
  OR2 : Logic  Operator=OR  IconShape=distinctive  AllPortsSameDT=off  OutDataTypeStr=boolean
  Selector : Selector  InputPortWidth=3  IndexOptions=Index vector (dialog)  Indices=2  OutputSizes=1
  Selector1 : Selector  InputPortWidth=3  IndexOptions=Index vector (dialog)  Indices=2  OutputSizes=1
  Subsystem3 : Subsystem
  Subsystem4 : Subsystem
  Sum1 : Sum
  Switch : Switch  Criteria=u2 > Threshold  SaturateOnIntegerOverflow=off  InputSameDT=off
  To Workspace2 : ToWorkspace  VariableName=TF_P  SampleTime=-1
  To Workspace3 : ToWorkspace  VariableName=Ang_312_P  SampleTime=-1
  To Workspace4 : ToWorkspace  VariableName=Ang_313_P  SampleTime=-1
  A_b/n : Outport
  Ang_312 : Outport  Port=2
  Ang_313 : Outport  Port=3
  T-F : Outport  Port=4
  wires:
  Constant5/1 -> GreaterThan/2
  [B] -> Subsystem4/1(angles313)
  Demux/2 -> Kinematics 313/2(wy), Kinematics 312/2(wy)  "wy"
  Sum1/1 -> Counter2/1
  From3/1 -> IC1/1
  OR2/1 -> Detect Rise Positive5/1  "singularity check 313"
  From/1 -> Selector/1
  Selector1/1 -> GreaterThan11/1, GreaterThan3/1, GreaterThan6/1, GreaterThan7/1  "prende solo theta 313"
  Constant/1 -> GreaterThan2/2
  GreaterThan6/1 -> AND1/2
  Constant6/1 -> GreaterThan5/2
  Subsystem4/1(angles312) -> IC2/1
  Counter2/1 -> Mod2/1
  Constant7/1 -> GreaterThan4/2
  IC1/1 -> Subsystem3/1(angles312)
  Constant19/1 -> GreaterThan7/2
  AND/1 -> OR1/1  "singularity check 312"
  Subsystem3/1(angles313) -> Kinematics 313/4(Input3)  "angles313"
  GreaterThan11/1 -> AND3/2
  AND1/1 -> OR2/1  "singularity chck 313"
  GreaterThan4/1 -> AND2/1
  Demux/3 -> Kinematics 313/3(wz), Kinematics 312/3(wz)  "wz"
  Detect Rise Positive5/1 -> Sum1/2
  Constant16/1 -> GreaterThan6/2
  IC2/1 -> Kinematics 312/4(Input3)
  GreaterThan2/1 -> AND/2
  Constant17/1 -> GreaterThan3/2
  Constant1/1 -> Mod2/2
  Selector/1 -> GreaterThan/1, GreaterThan2/1, GreaterThan5/1, GreaterThan4/1  "solo theta 312"
  GreaterThan7/1 -> AND3/1
  NOT2/1 -> T-F/1, To Workspace2/1, Switch/2, Kinematics 312/5(Logic), Kinematics 312/Enable
  OR1/1 -> Detect Rise Positive4/1
  GreaterThan3/1 -> AND1/1
  Constant18/1 -> GreaterThan11/2
  GreaterThan/1 -> AND/1
  Demux/1 -> Kinematics 313/1(wx), Kinematics 312/1(wx)  "wx"
  AND2/1 -> OR1/2  "singularity check 312"
  AND3/1 -> OR2/2  "singularity check 312"
  [B] -> Selector1/1
  Mod2/1 -> Kinematics 313/Enable, Kinematics 313/5(Logic), NOT2/1
  Kinematics 312/2(Output1) -> Switch/1
  GreaterThan5/1 -> AND2/2
  Detect Rise Positive4/1 -> Sum1/1
  w_b/1 -> Demux/1
  Switch/1 -> A_b/n/1
  Kinematics 313/3(Output1) -> Switch/3
  Kinematics 312/1(Output) -> To Workspace3/1, Ang_312/1
  Kinematics 313/1(Output) -> To Workspace4/1, Ang_313/1

== system Nadir_Pointing/Kinematics/Subsystem ==
  Ang_312 : Inport
  Ang_313 : Inport  Port=2
  T-F : Inport  Port=3
  Constant : Constant
  Constant1 : Constant  Value=0
  Constant2 : Constant
  Constant3 : Constant  Value=0
  Gain : Gain  Gain=-1
  Subsystem : Subsystem
  Subsystem4 : Subsystem
  Switch : Switch  Criteria=u2 > Threshold  SaturateOnIntegerOverflow=off  InputSameDT=off
  Switch1 : Switch  SaturateOnIntegerOverflow=off  InputSameDT=off
  To Workspace : ToWorkspace  VariableName=Ang_312_into_312_P  SampleTime=-1
  To Workspace1 : ToWorkspace  VariableName=Ang_313_into_312_P  SampleTime=-1
  wires:
  Constant/1 -> Switch/1
  Constant1/1 -> Switch/3
  Ang_312/1 -> Subsystem/1(Ang_312)
  Switch/1 -> Subsystem/Enable
  Subsystem/1(Ang312) -> To Workspace/1
  Gain/1 -> Switch1/2
  T-F/1 -> Gain/1, Switch/2
  Constant2/1 -> Switch1/1
  Constant3/1 -> Switch1/3
  Switch1/1 -> Subsystem4/Enable
  Subsystem4/1(angles312) -> To Workspace1/1
  Ang_313/1 -> Subsystem4/1(angles313)

== system Nadir_Pointing/M disturbances/M of B ==
  A b/n : Inport
  r_n : Inport  Port=2
  "B field " : Subsystem
  Cross Product : matrix_library/Cross Product
  Induction current : Constant  Value=jb
  M B : Outport
  wires:
  Cross Product/1 -> M B/1
  A b/n/1 -> "B field "/1(A b/n)
  "B field "/1(b_b) -> Cross Product/2
  Induction current/1 -> Cross Product/1
  r_n/1 -> "B field "/2(r_n)

== system Nadir_Pointing/M disturbances/M of G G ==
  Ab/l : Inport
  Constant1 : Constant  Value=I_tot
  Cross Product : matrix_library/Cross Product
  "D.C. of R " : Subsystem
  Gain : Gain  Gain=3
  Mean Angular Speed : Constant  Value=n
  Product1 : Product  Multiplication=Matrix(*)
  Product2 : Product
  Square : Math  Operator=square
  M_G_G : Outport
  wires:
  Mean Angular Speed/1 -> Square/1
  Square/1 -> Gain/1
  Product1/1 -> Cross Product/2
  Ab/l/1 -> "D.C. of R "/1(Ab/l)
  "D.C. of R "/1(c) -> Product1/2, Cross Product/1  "c"
  Gain/1 -> Product2/2  "3*n^2"
  Product2/1 -> M_G_G/1
  Constant1/1 -> Product1/1
  Cross Product/1 -> Product2/1

== system Nadir_Pointing/Sensors/Gyroscopic Sensor ==
  w_b/n : Inport
  Band-Limited White Noise : simulink/Sources/Band-Limited White Noise  Cov=[ARW]  Ts=n_t  seed=[23341]
  Band-Limited White Noise1 : simulink/Sources/Band-Limited White Noise  Cov=[RRW]  Ts=n_t  seed=[23341]
  Constant : Constant  Value=Miss_G
  Constant1 : Constant  Value=eye(3,3)
  Constant2 : Constant  Value=Gain_G
  Discrete-Time Integrator : DiscreteIntegrator  SampleTime=-1  ICPrevOutput=DiscIntNeverNeededParam  ICPrevScaledInput=DiscIntNeverNeededParam
  Product : Product  Inputs=3  Multiplication=Matrix(*)
  Product1 : Product
  Quantizer : Quantizer  QuantizationInterval=Gs_res
  Random Number : RandomNumber  Mean=1  Variance=0.0005  SampleTime=n_t
  Skew : Subsystem
  Sum : Sum  Inputs=|+|+||+
  Sum1 : Sum  Inputs=||+||-||
  Transpose : Math  Operator=transpose
  Zero-Order Hold : ZeroOrderHold  SampleTime=samp_t
  w_b/n_m : Outport
  wires:
  Band-Limited White Noise1/1 -> Discrete-Time Integrator/1
  Band-Limited White Noise/1 -> Sum/2
  Constant2/1 -> Product1/1
  Random Number/1 -> Product1/2
  Product1/1 -> Product/1
  Product/1 -> Sum/1
  Sum/1 -> Quantizer/1
  w_b/n/1 -> Zero-Order Hold/1
  Transpose/1 -> Product/2
  Zero-Order Hold/1 -> Product/3
  Sum1/1 -> Transpose/1
  Discrete-Time Integrator/1 -> Sum/3
  Constant1/1 -> Sum1/1
  Skew/1(Skew_Theta) -> Sum1/2
  Constant/1 -> Skew/1(Theta)
  Quantizer/1 -> w_b/n_m/1

== system Nadir_Pointing/Sensors/Horizon Sensor1 ==
  r_b : Inport
  Asin : Trigonometry  Operator=asin
  Atan2 : Trigonometry  Operator=atan2
  Band-Limited White Noise : simulink/Sources/Band-Limited White Noise  Cov=Hs_var  Ts=n_t  seed=[23341]
  Band-Limited White Noise1 : simulink/Sources/Band-Limited White Noise  Cov=Hs_var  Ts=n_t  seed=[23341]
  Cos : Trigonometry  Operator=cos
  Cos1 : Trigonometry  Operator=cos
  Demux : Demux  Outputs=3
  Mux : Mux  Inputs=3
  Product2 : Product
  Product3 : Product
  Quantizer : Quantizer  QuantizationInterval=Hs_res
  Quantizer1 : Quantizer  QuantizationInterval=Hs_res
  Sin : Trigonometry
  Sin1 : Trigonometry
  Sum1 : Sum  Inputs=|++
  Sum2 : Sum  Inputs=|++
  Zero-Order Hold : ZeroOrderHold  SampleTime=samp_t
  r_b_m : Outport
  wires:
  Mux/1 -> r_b_m/1
  Atan2/1 -> Sum1/1  "alpha"
  Demux/1 -> Atan2/2
  Product2/1 -> Mux/1  "rxm"
  Demux/2 -> Atan2/1  "ry"
  Asin/1 -> Sum2/1  "delta"
  Demux/3 -> Asin/1  "rz"
  Sin/1 -> Mux/3  "rzm"
  Band-Limited White Noise/1 -> Sum1/2
  Sum2/1 -> Quantizer/1
  Band-Limited White Noise1/1 -> Sum2/2
  Sum1/1 -> Quantizer1/1
  Sin1/1 -> Product3/1
  Cos/1 -> Product2/2, Product3/2
  Cos1/1 -> Product2/1
  Product3/1 -> Mux/2  "rym"
  Quantizer1/1 -> Sin1/1, Cos1/1
  Quantizer/1 -> Sin/1, Cos/1
  Zero-Order Hold/1 -> Demux/1
  r_b/1 -> Zero-Order Hold/1

== system Nadir_Pointing/Sensors/Sun Sensor1 ==
  S_b : Inport
  Asin : Trigonometry  Operator=asin
  Atan2 : Trigonometry  Operator=atan2
  Band-Limited White Noise : simulink/Sources/Band-Limited White Noise  Cov=Ss_var  Ts=n_t  seed=[23341]
  Band-Limited White Noise1 : simulink/Sources/Band-Limited White Noise  Cov=Ss_var  Ts=n_t  seed=[23341]
  Cos : Trigonometry  Operator=cos
  Cos1 : Trigonometry  Operator=cos
  Demux : Demux  Outputs=3
  Mux : Mux  Inputs=3
  Product2 : Product
  Product3 : Product
  Quantizer : Quantizer  QuantizationInterval=Ss_res
  Quantizer1 : Quantizer  QuantizationInterval=Ss_res
  Sin : Trigonometry
  Sin1 : Trigonometry
  Sum1 : Sum  Inputs=|++
  Sum2 : Sum  Inputs=|++
  Zero-Order Hold : ZeroOrderHold  SampleTime=samp_t
  S_b_m : Outport
  wires:
  Cos1/1 -> Product2/1
  S_b/1 -> Zero-Order Hold/1
  Sin1/1 -> Product3/1
  Sin/1 -> Mux/3  "rzm"
  Zero-Order Hold/1 -> Demux/1
  Mux/1 -> S_b_m/1
  Cos/1 -> Product2/2, Product3/2
  Product3/1 -> Mux/2  "rym"
  Sum1/1 -> Quantizer1/1
  Band-Limited White Noise/1 -> Sum1/2
  Sum2/1 -> Quantizer/1
  Band-Limited White Noise1/1 -> Sum2/2
  Demux/2 -> Atan2/1  "ry"
  Demux/3 -> Asin/1  "rz"
  Asin/1 -> Sum2/1  "delta"
  Demux/1 -> Atan2/2
  Atan2/1 -> Sum1/1  "alpha"
  Product2/1 -> Mux/1  "rxm"
  Quantizer/1 -> Sin/1, Cos/1
  Quantizer1/1 -> Sin1/1, Cos1/1

== system Nadir_Pointing/CMG/A/A2 rot ==
  angle : Inport
  Constant5 : Constant  Value=[0 0 0; 0 1 0; 0 0 0]
  Constant6 : Constant  Value=[1 0 0; 0 0 0; 0 0 1]
  Constant7 : Constant  Value=[0 0 1; 0 0 0; -1 0 0]
  Cos4 : Trigonometry  Operator=cos
  Product2 : Product
  Product3 : Product
  Sin4 : Trigonometry
  Sum : Sum  Inputs=|+||+||+
  A2 : Outport
  wires:
  Cos4/1 -> Product2/1
  Product2/1 -> Sum/2
  Constant7/1 -> Product3/2
  Sum/1 -> A2/1
  angle/1 -> Sin4/1, Cos4/1
  Constant6/1 -> Product2/2
  Sin4/1 -> Product3/1
  Product3/1 -> Sum/3
  Constant5/1 -> Sum/1

== system Nadir_Pointing/CMG/A/A2 rot1 ==
  angle : Inport
  Constant5 : Constant  Value=[0 0 0; 0 1 0; 0 0 0]
  Constant6 : Constant  Value=[1 0 0; 0 0 0; 0 0 1]
  Constant7 : Constant  Value=[0 0 1; 0 0 0; -1 0 0]
  Cos4 : Trigonometry  Operator=cos
  Product2 : Product
  Product3 : Product
  Sin4 : Trigonometry
  Sum : Sum  Inputs=|+||+||+
  A2 : Outport
  wires:
  Cos4/1 -> Product2/1
  Product2/1 -> Sum/2
  Constant7/1 -> Product3/2
  Sum/1 -> A2/1
  angle/1 -> Sin4/1, Cos4/1
  Constant6/1 -> Product2/2
  Sin4/1 -> Product3/1
  Product3/1 -> Sum/3
  Constant5/1 -> Sum/1

== system Nadir_Pointing/CMG/A/A3 rot ==
  angle : Inport
  Constant1 : Constant  Value=[0 0 0; 0 0 0; 0 0 1]
  Constant2 : Constant  Value=[1 0 0; 0 1 0; 0 0 0]
  Constant3 : Constant  Value=[0 1 0; -1 0 0; 0 0 0]
  Cos : Trigonometry  Operator=cos
  Product : Product
  Product1 : Product
  Sin : Trigonometry
  Sum : Sum  Inputs=|+||+||+
  A3 : Outport
  wires:
  Constant2/1 -> Product/2
  Sum/1 -> A3/1
  angle/1 -> Sin/1, Cos/1
  Product/1 -> Sum/2
  Cos/1 -> Product/1
  Sin/1 -> Product1/1
  Constant3/1 -> Product1/2
  Constant1/1 -> Sum/1
  Product1/1 -> Sum/3

== system Nadir_Pointing/CMG/A/A3 rot1 ==
  angle : Inport
  Constant1 : Constant  Value=[0 0 0; 0 0 0; 0 0 1]
  Constant2 : Constant  Value=[1 0 0; 0 1 0; 0 0 0]
  Constant3 : Constant  Value=[0 1 0; -1 0 0; 0 0 0]
  Cos : Trigonometry  Operator=cos
  Product : Product
  Product1 : Product
  Sin : Trigonometry
  Sum : Sum  Inputs=|+||+||+
  A3 : Outport
  wires:
  Constant2/1 -> Product/2
  Sum/1 -> A3/1
  angle/1 -> Sin/1, Cos/1
  Product/1 -> Sum/2
  Cos/1 -> Product/1
  Sin/1 -> Product1/1
  Constant3/1 -> Product1/2
  Constant1/1 -> Sum/1
  Product1/1 -> Sum/3

== system Nadir_Pointing/CMG/B/A2 rot ==
  angle : Inport
  Constant5 : Constant  Value=[0 0 0; 0 1 0; 0 0 0]
  Constant6 : Constant  Value=[1 0 0; 0 0 0; 0 0 1]
  Constant7 : Constant  Value=[0 0 1; 0 0 0; -1 0 0]
  Cos4 : Trigonometry  Operator=cos
  Product2 : Product
  Product3 : Product
  Sin4 : Trigonometry
  Sum : Sum  Inputs=|+||+||+
  A2 : Outport
  wires:
  Cos4/1 -> Product2/1
  Product2/1 -> Sum/2
  Constant7/1 -> Product3/2
  Sum/1 -> A2/1
  angle/1 -> Sin4/1, Cos4/1
  Constant6/1 -> Product2/2
  Sin4/1 -> Product3/1
  Product3/1 -> Sum/3
  Constant5/1 -> Sum/1

== system Nadir_Pointing/CMG/B/A2 rot1 ==
  angle : Inport
  Constant5 : Constant  Value=[0 0 0; 0 1 0; 0 0 0]
  Constant6 : Constant  Value=[1 0 0; 0 0 0; 0 0 1]
  Constant7 : Constant  Value=[0 0 1; 0 0 0; -1 0 0]
  Cos4 : Trigonometry  Operator=cos
  Product2 : Product
  Product3 : Product
  Sin4 : Trigonometry
  Sum : Sum  Inputs=|+||+||+
  A2 : Outport
  wires:
  Cos4/1 -> Product2/1
  Product2/1 -> Sum/2
  Constant7/1 -> Product3/2
  Sum/1 -> A2/1
  angle/1 -> Sin4/1, Cos4/1
  Constant6/1 -> Product2/2
  Sin4/1 -> Product3/1
  Product3/1 -> Sum/3
  Constant5/1 -> Sum/1

== system Nadir_Pointing/CMG/B/A3 rot ==
  angle : Inport
  Constant1 : Constant  Value=[0 0 0; 0 0 0; 0 0 1]
  Constant2 : Constant  Value=[1 0 0; 0 1 0; 0 0 0]
  Constant3 : Constant  Value=[0 1 0; -1 0 0; 0 0 0]
  Cos : Trigonometry  Operator=cos
  Product : Product
  Product1 : Product
  Sin : Trigonometry
  Sum : Sum  Inputs=|+||+||+
  A3 : Outport
  wires:
  Constant2/1 -> Product/2
  Sum/1 -> A3/1
  angle/1 -> Sin/1, Cos/1
  Product/1 -> Sum/2
  Cos/1 -> Product/1
  Sin/1 -> Product1/1
  Constant3/1 -> Product1/2
  Constant1/1 -> Sum/1
  Product1/1 -> Sum/3

== system Nadir_Pointing/CMG/B/A3 rot1 ==
  angle : Inport
  Constant1 : Constant  Value=[0 0 0; 0 0 0; 0 0 1]
  Constant2 : Constant  Value=[1 0 0; 0 1 0; 0 0 0]
  Constant3 : Constant  Value=[0 1 0; -1 0 0; 0 0 0]
  Cos : Trigonometry  Operator=cos
  Product : Product
  Product1 : Product
  Sin : Trigonometry
  Sum : Sum  Inputs=|+||+||+
  A3 : Outport
  wires:
  Constant2/1 -> Product/2
  Sum/1 -> A3/1
  angle/1 -> Sin/1, Cos/1
  Product/1 -> Sum/2
  Cos/1 -> Product/1
  Sin/1 -> Product1/1
  Constant3/1 -> Product1/2
  Constant1/1 -> Sum/1
  Product1/1 -> Sum/3

== system Nadir_Pointing/CMG/Singularity Condition/Normalization1 ==
  v : Inport
  Divide : Product  Inputs=*/
  Dot Product : DotProduct  OutDataTypeStr=Inherit: Inherit via internal rule
  Square Root : Sqrt
  v^ : Outport
  wires:
  Divide/1 -> v^/1
  Dot Product/1 -> Square Root/1
  v/1 -> Divide/1, Dot Product/2, Dot Product/1
  Square Root/1 -> Divide/2

== system Nadir_Pointing/CMG/Singularity Condition/Subsystem ==
  In1 : Inport
  Enable : EnablePort
  Constant : Constant  Value=[0;0;0]
  MATLAB Function : MATLAB Function  TreatAsAtomicUnit=on
  Product : Product  Multiplication=Matrix(*)
  Delta_dot_n : Outport
  wires:
  MATLAB Function/1(y) -> Product/1
  Product/1 -> Delta_dot_n/1
  In1/1 -> MATLAB Function/1(B)
  Constant/1 -> Product/2

== system Nadir_Pointing/Control/Linear and Non linear control/Skew ==
  w_err : Inport
  Constant1 : Constant  Value=[1;0;0]
  Constant2 : Constant  Value=[0;1;0]
  Constant3 : Constant  Value=[0;0;1]
  Cross Product : matrix_library/Cross Product
  Cross Product1 : matrix_library/Cross Product
  Cross Product2 : matrix_library/Cross Product
  Display : Display
  Matrix Concatenate : Concatenate  NumInputs=3  Mode=Multidimensional array  ConcatenateDimension=2
  Skew_w_err : Outport
  wires:
  Cross Product/1 -> Matrix Concatenate/1
  Constant3/1 -> Cross Product2/2
  Constant1/1 -> Cross Product/2
  Cross Product1/1 -> Matrix Concatenate/2
  Matrix Concatenate/1 -> Display/1, Skew_w_err/1
  w_err/1 -> Cross Product1/1, Cross Product2/1, Cross Product/1
  Cross Product2/1 -> Matrix Concatenate/3
  Constant2/1 -> Cross Product1/2

== system Nadir_Pointing/Control/Target Model/Subsystem ==
  True Anomaly0 : Inport
  Constant : Constant
  Constant1 : Constant
  Constant5 : Constant  Value=3/2
  Cos1 : Trigonometry  Operator=cos
  Discrete-Time Integrator : DiscreteIntegrator  InitialConditionSource=external  SampleTime=-1  ICPrevOutput=DiscIntNeverNeededParam  ICPrevScaledInput=DiscIntNeverNeededParam
  Divide1 : Product  Inputs=*/
  Earth rotation rate : Gain  Gain=we
  Eccentricity : Constant  Value=e
  Gain : Gain  Gain=e
  Power : Math  Operator=pow
  Square : Math  Operator=square
  Square1 : Math  Operator=square
  Sum2 : Sum  Inputs=|++
  Sum3 : Sum  Inputs=|+-
  theta : Outport
  teta_dot : Outport  Port=2
  wires:
  Constant/1 -> Sum2/1
  Eccentricity/1 -> Square/1
  Sum3/1 -> Power/1
  Divide1/1 -> Discrete-Time Integrator/1, teta_dot/1
  Cos1/1 -> Gain/1
  Sum2/1 -> Square1/1
  True Anomaly0/1 -> Discrete-Time Integrator/2
  Power/1 -> Divide1/2
  Constant1/1 -> Sum3/1
  Square1/1 -> Earth rotation rate/1
  Constant5/1 -> Power/2
  Discrete-Time Integrator/1 -> theta/1, Cos1/1  "theta"
  Earth rotation rate/1 -> Divide1/1
  Gain/1 -> Sum2/2
  Square/1 -> Sum3/2

== system Nadir_Pointing/Control/Target Model/Subsystem1 ==
  OM : Inport
  i : Inport  Port=2
  w+f : Inport  Port=3
  2 A1 rot : Subsystem
  2 A3 rot : Subsystem
  2 A3 rot2 : Subsystem
  Product : Product  Inputs=3  Multiplication=Matrix(*)
  A313 : Outport
  wires:
  2 A3 rot/1(A23) -> Product/3
  OM/1 -> 2 A3 rot/1(ang)
  Product/1 -> A313/1
  2 A1 rot/1(A21) -> Product/2
  2 A3 rot2/1(A233) -> Product/1
  w+f/1 -> 2 A3 rot2/1(ang)
  i/1 -> 2 A1 rot/1(ang)

== system Nadir_Pointing/Environment/A l//n for elliptical orbit/Subsystem ==
  True Anomaly0 : Inport
  Constant : Constant
  Constant1 : Constant
  Constant5 : Constant  Value=3/2
  Cos1 : Trigonometry  Operator=cos
  Divide1 : Product  Inputs=*/
  Earth rotation rate : Gain  Gain=we
  Eccentricity : Constant  Value=e
  Gain : Gain  Gain=e
  Integrator : Integrator  InitialConditionSource=external
  Power : Math  Operator=pow
  Square : Math  Operator=square
  Square1 : Math  Operator=square
  Sum2 : Sum  Inputs=|++
  Sum3 : Sum  Inputs=|+-
  theta : Outport
  teta_dot : Outport  Port=2
  wires:
  Constant/1 -> Sum2/1
  Eccentricity/1 -> Square/1
  Sum3/1 -> Power/1
  Divide1/1 -> teta_dot/1, Integrator/1
  Cos1/1 -> Gain/1
  Sum2/1 -> Square1/1
  True Anomaly0/1 -> Integrator/2
  Power/1 -> Divide1/2
  Constant1/1 -> Sum3/1
  Square1/1 -> Earth rotation rate/1
  Constant5/1 -> Power/2
  Integrator/1 -> theta/1, Cos1/1  "theta"
  Earth rotation rate/1 -> Divide1/1
  Gain/1 -> Sum2/2
  Square/1 -> Sum3/2

== system Nadir_Pointing/Environment/A l//n for elliptical orbit/Subsystem1 ==
  OM : Inport
  i : Inport  Port=2
  w+f : Inport  Port=3
  2 A1 rot : Subsystem
  2 A3 rot : Subsystem
  2 A3 rot2 : Subsystem
  Product : Product  Inputs=3  Multiplication=Matrix(*)
  A313 : Outport
  wires:
  2 A3 rot/1(A23) -> Product/3
  OM/1 -> 2 A3 rot/1(ang)
  Product/1 -> A313/1
  2 A1 rot/1(A21) -> Product/2
  2 A3 rot2/1(A233) -> Product/1
  w+f/1 -> 2 A3 rot2/1(ang)
  i/1 -> 2 A1 rot/1(ang)

== system Nadir_Pointing/Environment/Kep 2bp/Subsystem ==
  OM : Inport
  i : Inport  Port=2
  w : Inport  Port=3
  2 A1 rot : Subsystem
  2 A3 rot : Subsystem
  2 A3 rot2 : Subsystem
  Product : Product  Inputs=3  Multiplication=Matrix(*)
  A313 : Outport
  wires:
  2 A3 rot/1(A23) -> Product/3
  OM/1 -> 2 A3 rot/1(angolo)
  Product/1 -> A313/1
  2 A1 rot/1(A21) -> Product/2
  2 A3 rot2/1(A233) -> Product/1
  w/1 -> 2 A3 rot2/1(angolo)
  i/1 -> 2 A1 rot/1(theta2)

== system Nadir_Pointing/Kinematics/Euler Angles/Kinematics 312 ==
  wx : Inport
  wy : Inport  Port=2
  wz : Inport  Port=3
  Input3 : Inport  Port=4
  Logic : Inport  Port=5
  Enable : EnablePort  StatesWhenEnabling=reset
  Demux : Demux  Outputs=3
  Demux1 : Demux  Outputs=3
  Goto : Goto  TagVisibility=global
  Integrator3 : Integrator  ExternalReset=rising  InitialConditionSource=external  ShowStatePort=on
  Matrix Multiply : Product  Inputs=3  Multiplication=Matrix(*)
  Mux : Mux  Inputs=3
  Mux1 : Mux  Inputs=3
  Subsystem1 : Subsystem
  Subsystem3 : Subsystem
  Subsystem4 : Subsystem
  Subsystem5 : Subsystem
  Subsystem7 : Subsystem
  Subsystem9 : Subsystem
  To Workspace1 : ToWorkspace  VariableName=A312_P  SampleTime=-1
  Output : Outport
  Output1 : Outport  Port=2
  wires:
  Integrator3/1 -> Demux/1
  Integrator3/State -> Goto/1
  Demux/1 -> Mux1/1  "phi312"
  Demux/2 -> Mux1/2, Subsystem1/2(theta), Subsystem3/3(theta)  "theta312"
  Demux/3 -> Mux1/3, Subsystem1/4(psi), Subsystem4/3(psi), Subsystem3/4(psi)  "psi312"
  wx/1 -> Subsystem3/1(wx), Subsystem4/1(wx), Subsystem1/1(wx)
  wz/1 -> Subsystem3/5(wz), Subsystem4/2(wz), Subsystem1/3(wz)
  wy/1 -> Subsystem3/2(wy)
  Subsystem1/1(Out1) -> Mux/1
  Subsystem4/1(Out1) -> Mux/2
  Subsystem3/1(Out1) -> Mux/3
  Mux/1 -> Integrator3/1
  Mux1/1 -> Demux1/1, Output/1  "angles312"
  Input3/1 -> Integrator3/3  "IC312"
  Logic/1 -> Integrator3/2
  Demux1/3 -> Subsystem5/1(psi312)
  Subsystem9/1(3) -> Matrix Multiply/3
  Subsystem5/1(2) -> Matrix Multiply/1
  Demux1/2 -> Subsystem7/1(theta312)
  Demux1/1 -> Subsystem9/1(phi312)
  Subsystem7/1(1) -> Matrix Multiply/2
  Matrix Multiply/1 -> Output1/1, To Workspace1/1  "A"

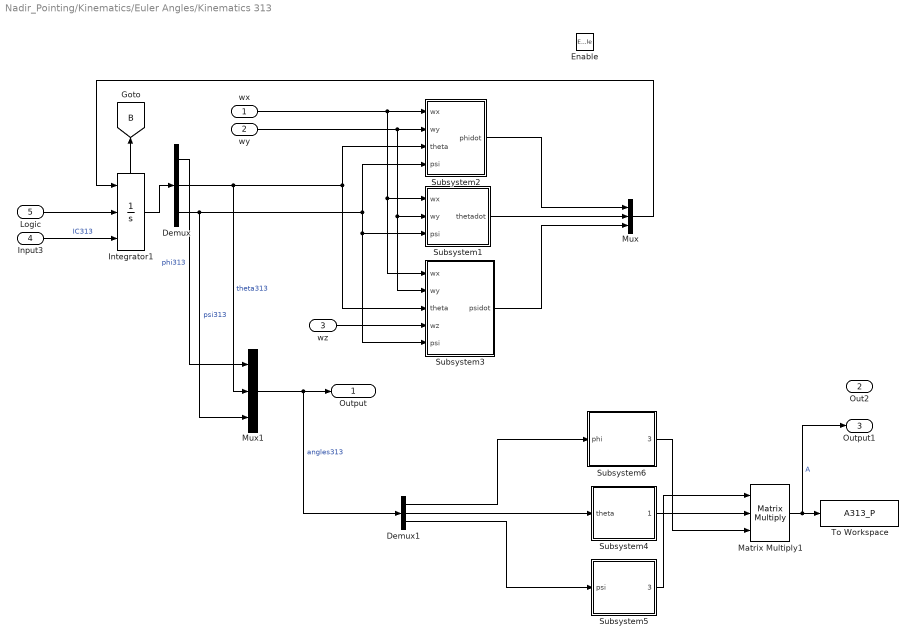
== system Nadir_Pointing/Kinematics/Euler Angles/Kinematics 313 ==
  wx : Inport
  wy : Inport  Port=2
  wz : Inport  Port=3
  Input3 : Inport  Port=4
  Logic : Inport  Port=5
  Enable : EnablePort  StatesWhenEnabling=reset
  Demux : Demux  Outputs=3
  Demux1 : Demux  Outputs=3
  Integrator1 : Integrator  ExternalReset=rising  InitialConditionSource=external  ShowStatePort=on
  Matrix Multiply1 : Product  Inputs=3  Multiplication=Matrix(*)
  Mux : Mux  Inputs=3
  Mux1 : Mux  Inputs=3
  Subsystem1 : Subsystem
  Subsystem2 : Subsystem
  Subsystem3 : Subsystem
  Subsystem4 : Subsystem
  Subsystem5 : Subsystem
  Subsystem6 : Subsystem
  To Workspace : ToWorkspace  VariableName=A313_P  SampleTime=-1
  Output : Outport
  Out2 : Outport  Port=2
  Output1 : Outport  Port=3
  tag scope: B=global
  wires:
  Integrator1/State -> [B]
  Integrator1/1 -> Demux/1
  Subsystem3/1(psidot) -> Mux/3
  Subsystem2/1(phidot) -> Mux/1
  Demux/1 -> Mux1/1  "phi313"
  Subsystem1/1(thetadot) -> Mux/2
  Mux/1 -> Integrator1/1
  Demux/2 -> Subsystem3/3(theta), Subsystem2/3(theta), Mux1/2  "theta313"
  Demux/3 -> Mux1/3, Subsystem1/3(psi), Subsystem3/5(psi), Subsystem2/4(psi)  "psi313"
  wx/1 -> Subsystem1/1(wx), Subsystem3/1(wx), Subsystem2/1(wx)
  wy/1 -> Subsystem3/2(wy), Subsystem1/2(wy), Subsystem2/2(wy)
  wz/1 -> Subsystem3/4(wz)
  Mux1/1 -> Demux1/1, Output/1  "angles313"
  Input3/1 -> Integrator1/3  "IC313"
  Logic/1 -> Integrator1/2
  Demux1/2 -> Subsystem4/1(theta)
  Subsystem5/1(3) -> Matrix Multiply1/1
  Subsystem4/1(1) -> Matrix Multiply1/2
  Demux1/3 -> Subsystem5/1(psi)
  Demux1/1 -> Subsystem6/1(phi)
  Subsystem6/1(3) -> Matrix Multiply1/3
  Matrix Multiply1/1 -> Output1/1, To Workspace/1  "A"

== system Nadir_Pointing/Kinematics/Euler Angles/Subsystem3 ==
  angles312 : Inport
  Subsystem10 : Subsystem
  Subsystem12 : Subsystem
  Subsystem4 : Subsystem
  Subsystem6 : Subsystem
  angles313 : Outport
  wires:
  Subsystem12/1(Out1) -> Subsystem4/1(matrix313)  "matrix313"
  angles312/1 -> Subsystem6/1(In1)
  Subsystem10/1(angles313) -> Subsystem12/1(angles313)  "angles313"
  Subsystem6/1(Out1) -> Subsystem10/1(In1)
  Subsystem4/1(angles313) -> angles313/1  "angles313"

== system Nadir_Pointing/Kinematics/Euler Angles/Subsystem4 ==
  angles313 : Inport
  Subsystem1 : Subsystem
  Subsystem12 : Subsystem
  angles312 : Outport
  wires:
  Subsystem12/1(Out1) -> Subsystem1/1(matrix313)  "matrix313"
  Subsystem1/1(angles312) -> angles312/1  "angles312"
  angles313/1 -> Subsystem12/1(angles313)

== system Nadir_Pointing/Kinematics/Subsystem/Subsystem ==
  Ang_312 : Inport
  Enable : EnablePort
  Ang312 : Outport
  wires:
  Ang_312/1 -> Ang312/1
